simulink model "HH"  (R2019a)
settings: Solver=VariableStepAuto  StartTime=0.0  StopTime=10.0  RelTol=1e-9
values from neighbouring files (symbols this model uses):
  C = 1    [H_H.m]
  E_k = -12    [H_H.m]
  E_L = 10.613    [H_H.m]
  E_na = 115    [H_H.m]
  G_k = 36    [H_H.m]
  G_L = 0.3    [H_H.m]
  G_na = 120    [H_H.m]
  H_init = .596    (= 0.596)    [H_H.m]
  I_stim = 10    [H_H.m]
  M_init = 5.296E-2    (= 0.05296)    [H_H.m]
  N_init = 0.3177    [H_H.m]
  V_init = 0    [H_H.m]
settings Model: Creator=Pranav Maddula  LastModifiedBy=Pranav Maddula

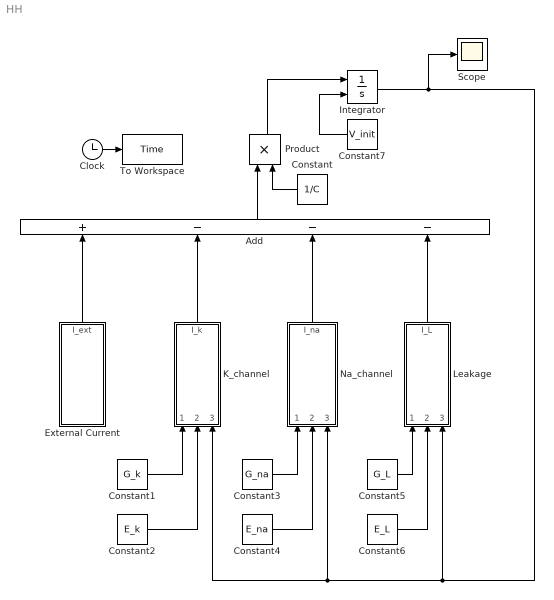
== system HH ==
  Add : Sum  Inputs=+---
  Clock : Clock
  Constant : Constant  Value=1/C
  Constant1 : Constant  Value=G_k
  Constant2 : Constant  Value=E_k
  Constant3 : Constant  Value=G_na
  Constant4 : Constant  Value=E_na
  Constant5 : Constant  Value=G_L
  Constant6 : Constant  Value=E_L
  Constant7 : Constant  Value=V_init
  External Current : Subsystem
  Integrator : Integrator  InitialConditionSource=external
  K_channel : Subsystem
  Leakage : Subsystem
  Na_channel : Subsystem
  Product : Product
  Scope : Scope
  To Workspace : ToWorkspace  VariableName=Time  SampleTime=-1
  wires:
  Clock/1 -> To Workspace/1
  External Current/1(I_ext) -> Add/1
  K_channel/1(I_k) -> Add/2
  Na_channel/1(I_na) -> Add/3
  Leakage/1(I_L) -> Add/4
  Add/1 -> Product/1
  Constant/1 -> Product/2
  Product/1 -> Integrator/1
  Integrator/1 -> Leakage/3(V_m), Na_channel/3(V_m), K_channel/3("V_m "), Scope/1
  Constant1/1 -> K_channel/1(G_k)
  Constant2/1 -> K_channel/2("E_k ")
  Constant3/1 -> Na_channel/1("G_na ")
  Constant4/1 -> Na_channel/2(E_na)
  Constant5/1 -> Leakage/1(G_L)
  Constant6/1 -> Leakage/2(E_L)
  Constant7/1 -> Integrator/2

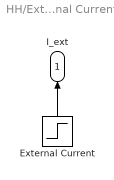
== system HH/External Current ==
  External Current : Step  After=I_stim  SampleTime=0
  I_ext : Outport
  wires:
  External Current/1 -> I_ext/1

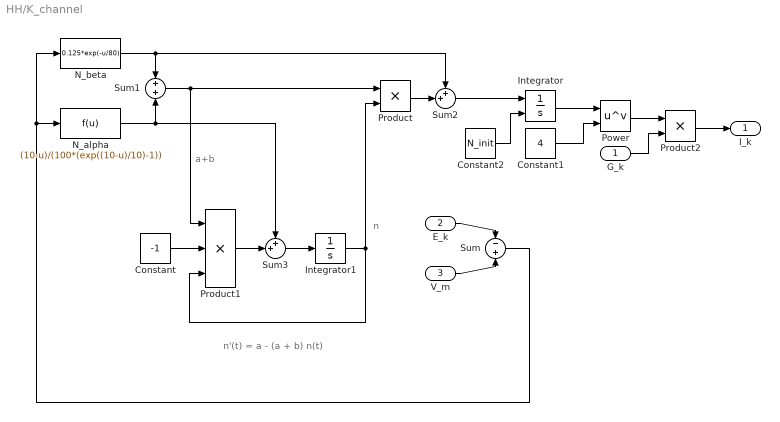
== system HH/K_channel ==
  note: a+b
  note: n
  note: n'(t) = a - (a + b) n(t)
  G_k : Inport
  "E_k " : Inport  Port=2
  "V_m " : Inport  Port=3
  Constant : Constant  Value=-1
  Constant1 : Constant  Value=4
  Constant2 : Constant  Value=N_init
  Integrator : Integrator  InitialConditionSource=external
  Integrator1 : Integrator
  N_alpha : Fcn  Expr=(10-u)/(100*(exp((10-u)/10)-1))
  N_beta : Fcn  Expr=0.125*exp(-u/80)
  Power : Math  Operator=pow  SaturateOnIntegerOverflow=on
  Product : Product
  Product1 : Product  Inputs=3
  Product2 : Product
  Sum : Sum  Inputs=-+
  Sum1 : Sum
  Sum2 : Sum  Inputs=++|
  Sum3 : Sum  Inputs=++|
  I_k : Outport
  wires:
  "E_k "/1 -> Sum/1
  "V_m "/1 -> Sum/2
  N_beta/1 -> Sum2/1, Sum1/1
  N_alpha/1 -> Sum3/1, Sum1/2
  Product/1 -> Sum2/2
  Sum2/1 -> Integrator/1
  Sum1/1 -> Product1/1, Product/1
  Constant/1 -> Product1/2
  Product1/1 -> Sum3/2
  Sum3/1 -> Integrator1/1
  Integrator1/1 -> Product/2, Product1/3
  Integrator/1 -> Power/1
  Constant1/1 -> Power/2
  Product2/1 -> I_k/1
  Power/1 -> Product2/1
  G_k/1 -> Product2/2
  Sum/1 -> N_beta/1, N_alpha/1
  Constant2/1 -> Integrator/2

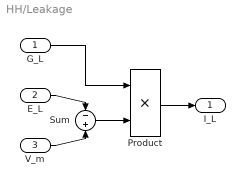
== system HH/Leakage ==
  G_L : Inport
  E_L : Inport  Port=2
  V_m : Inport  Port=3
  Product : Product
  Sum : Sum  Inputs=-+
  I_L : Outport
  wires:
  E_L/1 -> Sum/1
  V_m/1 -> Sum/2
  Sum/1 -> Product/2
  G_L/1 -> Product/1
  Product/1 -> I_L/1

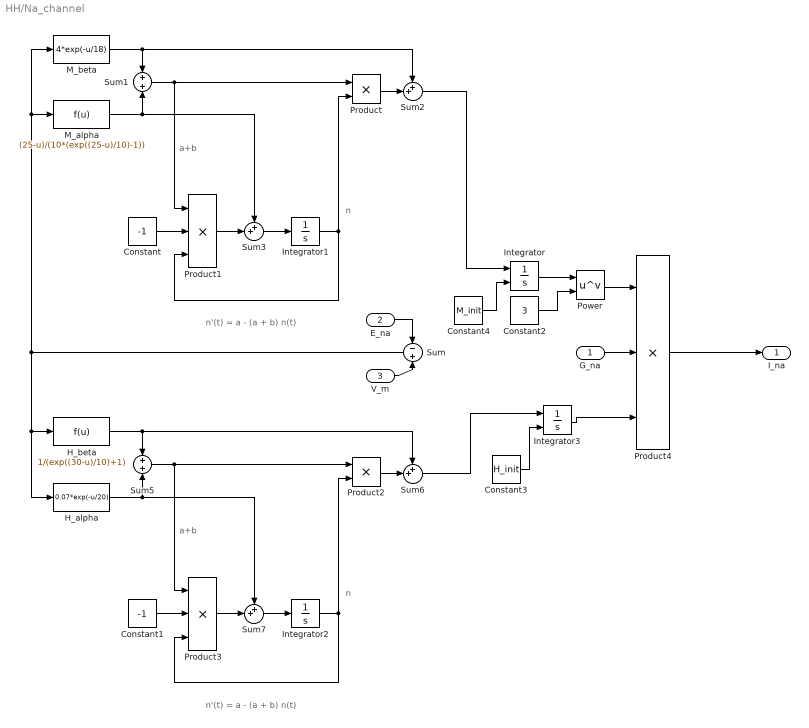
== system HH/Na_channel ==
  note: a+b
  note: n'(t) = a - (a + b) n(t)
  note: n
  note: n'(t) = a - (a + b) n(t)
  note: a+b
  note: n
  "G_na " : Inport
  E_na : Inport  Port=2
  V_m : Inport  Port=3
  Constant : Constant  Value=-1
  Constant1 : Constant  Value=-1
  Constant2 : Constant  Value=3
  Constant3 : Constant  Value=H_init
  Constant4 : Constant  Value=M_init
  H_alpha : Fcn  Expr=0.07*exp(-u/20)
  H_beta : Fcn  Expr=1/(exp((30-u)/10)+1)
  Integrator : Integrator  InitialConditionSource=external
  Integrator1 : Integrator
  Integrator2 : Integrator
  Integrator3 : Integrator  InitialConditionSource=external
  M_alpha : Fcn  Expr=(25-u)/(10*(exp((25-u)/10)-1))
  M_beta : Fcn  Expr=4*exp(-u/18)
  Power : Math  Operator=pow  SaturateOnIntegerOverflow=on
  Product : Product
  Product1 : Product  Inputs=3
  Product2 : Product
  Product3 : Product  Inputs=3
  Product4 : Product  Inputs=3
  Sum : Sum  Inputs=-+
  Sum1 : Sum
  Sum{2..3,6..7} (4 alike) : Sum  Inputs=++|
  Sum5 : Sum
  I_na : Outport
  wires:
  M_beta/1 -> Sum2/1, Sum1/1
  Sum/1 -> M_beta/1, M_alpha/1, H_alpha/1, H_beta/1
  M_alpha/1 -> Sum3/1, Sum1/2
  Sum1/1 -> Product1/1, Product/1
  Constant/1 -> Product1/2
  Sum3/1 -> Integrator1/1
  V_m/1 -> Sum/2
  Integrator1/1 -> Product/2, Product1/3
  Product/1 -> Sum2/2
  Product1/1 -> Sum3/2
  E_na/1 -> Sum/1
  Sum7/1 -> Integrator2/1
  Product3/1 -> Sum7/2
  Integrator2/1 -> Product2/2, Product3/3
  Product2/1 -> Sum6/2
  Constant1/1 -> Product3/2
  Sum5/1 -> Product3/1, Product2/1
  H_beta/1 -> Sum6/1, Sum5/1
  H_alpha/1 -> Sum7/1, Sum5/2
  Product4/1 -> I_na/1
  Constant2/1 -> Power/2
  Integrator/1 -> Power/1
  Sum2/1 -> Integrator/1
  Power/1 -> Product4/1
  "G_na "/1 -> Product4/2
  Integrator3/1 -> Product4/3
  Sum6/1 -> Integrator3/1
  Constant3/1 -> Integrator3/2
  Constant4/1 -> Integrator/2
